simulink model "QuadrotorSimControl"  (R2025a)
settings: Solver=VariableStepAuto  StartTime=0.0  StopTime=50  RelTol=1e-3
libraries: sharedtransform x1
settings Model: Creator=User  LastModifiedBy=luke

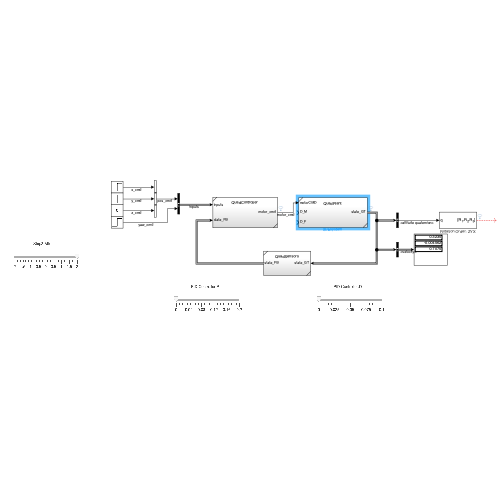
[thumbnail: Simulink's stored preview of the top-level diagram]
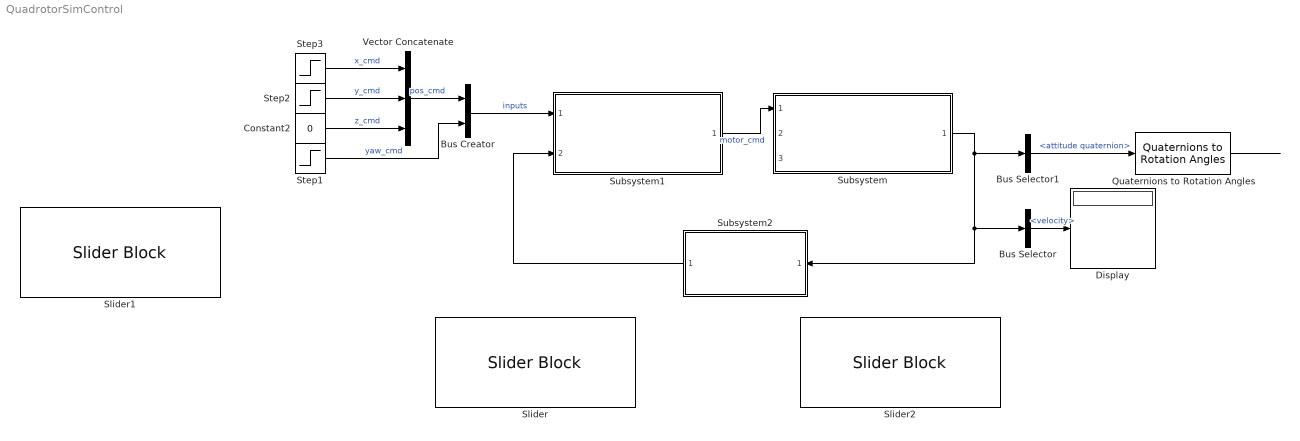
== system QuadrotorSimControl ==
  Bus Creator : BusCreator  Inputs=2
  Bus Selector : BusSelector  OutputSignals=Translation State.velocity
  Bus Selector1 : BusSelector  OutputSignals=Attitude State.attitude quaternion
  Constant2 : Constant  Value=0
  Display : Display
  Quaternions to Rotation Angles : sharedtransform/Quaternions to Rotation Angles  rotationOrder=ZYX  aMode=aMode
  Slider : SliderBlock  ScaleMax=0.2
  Slider1 : SliderBlock  ScaleMin=-2  ScaleMax=2
  Slider2 : SliderBlock  ScaleMax=0.1
  Step1 : Step  Time=5  After=0  SampleTime=0
  Step2 : Step  Time=5  After=0  SampleTime=0
  Step3 : Step  Time=5  After=2  SampleTime=0
  Subsystem : Subsystem  ReferencedSubsystem=QuadPlant
  Subsystem1 : Subsystem  ReferencedSubsystem=QuadController
  Subsystem2 : Subsystem  ReferencedSubsystem=QuadSensors
  Vector Concatenate : Concatenate  NumInputs=3
  wires:
  Subsystem/1 -> Bus Selector/1, Subsystem2/1, Bus Selector1/1
  Subsystem2/1 -> Subsystem1/2
  Subsystem1/1 -> Subsystem/1  "motor_cmd"
  Step3/1 -> Vector Concatenate/1  "x_cmd"
  Step2/1 -> Vector Concatenate/2  "y_cmd"
  Step1/1 -> Bus Creator/2  "yaw_cmd"
  Constant2/1 -> Vector Concatenate/3  "z_cmd"
  Vector Concatenate/1 -> Bus Creator/1  "pos_cmd"
  Bus Creator/1 -> Subsystem1/1  "inputs"
  Bus Selector/1 -> Display/1  "<velocity>"
  Bus Selector1/1 -> Quaternions to Rotation Angles/1  "<attitude quaternion>"
  Quaternions to Rotation Angles/1 -> ?
